simulink model "lfsr_test"  (R2021b)
settings: Solver=FixedStepAuto  StartTime=0.0  StopTime=10e-3  RelTol=1e-3
undefined symbols (not defined in the file or in its folder): hw, xc7z020clg400
libraries: hdlBasic x13, simulink x1, vmcUtilities x1
settings Model: Creator=berndorfer  LastModifiedBy=berndorfer

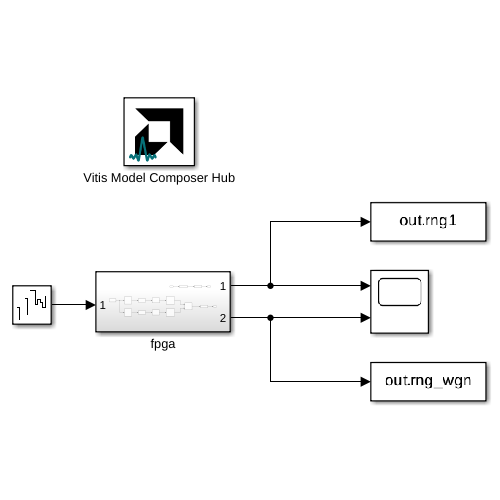
[thumbnail: Simulink's stored preview of the top-level diagram]
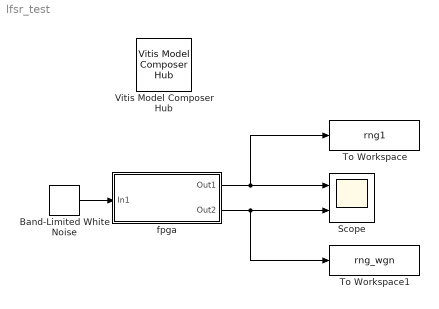
== system lfsr_test ==
  Band-Limited White Noise : simulink/Sources/Band-Limited White Noise  Cov=[2 * hw.t_s * hw.oversample]  Ts=hw.t_s*hw.oversample  seed=[23341]
  Scope : Scope  NumInputPorts=2
  To Workspace : ToWorkspace  VariableName=rng1  SaveFormat=Timeseries  SampleTime=-1
  To Workspace1 : ToWorkspace  VariableName=rng_wgn  SaveFormat=Timeseries  SampleTime=-1
  Vitis Model Composer Hub : vmcUtilities/Vitis Model Composer Hub  Tag=genX  CodeGeneration=off  SubsystemName=fpga  TargetDirectory=./code  ExportType=AI Engines  IpVendor=xilinx.com  IpLibrary=hls  IpVersion=1.0  IpHWLanguage=Verilog  AieCompilerOptions={}  AieSimulatorOptions={}  CreateTestbench=off  TestbenchStackSize=10  RunRtlSim=off  RunCSim=off  RunAieSim=off  AieSimTimeout=50000  RunAieSimProfiling=off  LaunchVitisAnalyzer=off  PlotOutput=off  RunX86Sim=off  X86SimTimeout=10  GenHwImage=off  GenLibadfXo=off  PlatformType=Not Specified  HwSystemType=Baremetal  HwValidationTarget=hw  ProjDevice=xc7z020clg400-1  ProjDevicePart=xc7z020clg400-1  AIEType=None  SamplePeriod=-1  ClockFrequency=200  DataPathParallelism=1  xilinxfamily=zynq  part=xc7z020  speed=-1  package=clg400  directory=./code/ip/fpga/src  testbench=off  incr_netlist=off  synthesis_tool=Vivado  clock_wrapper=Clock Enables  dbl_ovrd=According to Block Masks  dcm_input_clock_period=10  sysclk_period=4  simulink_period=4e-9  eval_field=0  LogFileName=''  NThreads=4
  fpga : Subsystem
  wires:
  fpga/1(Out1) -> Scope/1, To Workspace/1
  Band-Limited White Noise/1 -> fpga/1(In1)
  fpga/2(Out2) -> Scope/2, To Workspace1/1

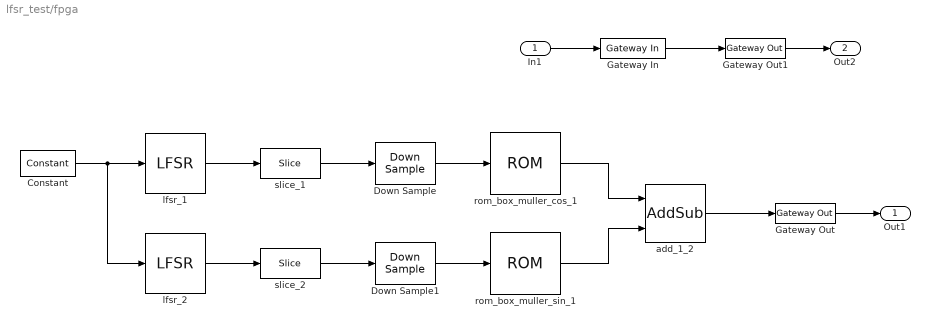
== system lfsr_test/fpga ==
  In1 : Inport
  Constant : hdlBasic/Constant  const=1.0  gui_display_data_type=Boolean  arith_type=Boolean  n_bits=16  bin_pt=14  preci_type=Single  exp_width=8  frac_width=24  explicit_period=on  period=hw.t_s*2  XmcBlockStatus=1  maskContainerNames=tabcontainer1  block_type=constant  block_config=sysgen:Constant_config
  Down Sample : hdlBasic/Down Sample  sample_ratio=hw.oversample/2  sample_phase="Last Value of Frame  (most efficient)"  en=off  rst=off  latency=1  XmcBlockStatus=1  maskContainerNames=group1  block_type=dsamp  block_config=sysgen:Downsample_config
  Down Sample1 : hdlBasic/Down Sample  sample_ratio=hw.oversample/2  sample_phase="Last Value of Frame  (most efficient)"  en=off  rst=off  latency=1  XmcBlockStatus=1  maskContainerNames=group1  block_type=dsamp  block_config=sysgen:Downsample_config
  Gateway In : hdlBasic/Gateway In  gui_display_data_type=Fixed-point  arith_type=Signed (2's comp)  n_bits=13  bin_pt=7  preci_type=Single  exp_width=8  frac_width=24  rows=1  columns=1  quantization=Truncate  overflow=Saturate  period=hw.t_s*hw.oversample  UseAsADC=off  ADCChannel='1'  interface=None  automatic_assignment=on  address_offset=hex2dec('00')  intf_name=''  intf_description=''  default_value=0  timing_constraint=None  locs_specified=off  LOCs={}  io_standard={}  inherit_from_input=off  hdl_port=on  XmcBlockStatus=1  maskContainerNames=group4  block_type=gatewayin  block_config=sysgen:gateway_in_config  block_width_w=590  block_height_w=620  block_width=640  block_height=850
  Gateway Out : hdlBasic/Gateway Out  inherit_from_input=off  hdl_port=on  rows=1  columns=1  UseAsDAC=off  DACChannel='1'  interface=None  automatic_assignment=on  address_offset=hex2dec('00')  intf_name=''  intf_description=''  timing_constraint=None  locs_specified=off  LOCs={}  io_standard={}  XmcBlockStatus=1  maskContainerNames=group4  block_type=gatewayout  block_config=sysgen:gateway_out_config  block_width_w=590  block_height_w=620  block_width=620  block_height=750
  Gateway Out1 : hdlBasic/Gateway Out  inherit_from_input=off  hdl_port=on  rows=1  columns=1  UseAsDAC=off  DACChannel='1'  interface=None  automatic_assignment=on  address_offset=hex2dec('00')  intf_name=''  intf_description=''  timing_constraint=None  locs_specified=off  LOCs={}  io_standard={}  XmcBlockStatus=1  maskContainerNames=group4  block_type=gatewayout  block_config=sysgen:gateway_out_config  block_width_w=590  block_height_w=620  block_width=620  block_height=750
  add_1_2 : hdlBasic/AddSub  mode=Addition  use_carryin=off  use_carryout=off  en=off  latency=1  precision=User Defined  arith_type="Signed  (2's comp)"  n_bits=13  bin_pt=7  quantization=Truncate  overflow=Wrap  use_behavioral_HDL=off  hw_selection=Fabric  pipelined=off  XmcBlockStatus=1  maskContainerNames=tabcontainer1  block_type=addsub  block_config=sysgen:Addsub_config
  lfsr_1 : hdlBasic/LFSR  lfsr_type=Galois  gate_type=XOR  n_bits=24  maxpolynomial=off  polynomial='c20001'  rst_value='927ce9'  rst=off  en=on  reloadable_seed=off  input_type=off  output_type=on  arith_type=Unsigned  bin_pt=0  explicit_period=off  period=1  XmcBlockStatus=1  maskContainerNames=tabcontainer1  block_type=lfsr  block_config=sysgen:LFSR_config
  lfsr_2 : hdlBasic/LFSR  lfsr_type=Galois  gate_type=XOR  n_bits=24  maxpolynomial=off  polynomial='c20001'  rst_value='6c6d84'  rst=off  en=on  reloadable_seed=off  input_type=off  output_type=on  arith_type=Unsigned  bin_pt=0  explicit_period=off  period=1  XmcBlockStatus=1  maskContainerNames=tabcontainer1  block_type=lfsr  block_config=sysgen:LFSR_config
  rom_box_muller_cos_1 : hdlBasic/ROM  depth=4096  initVector=ip.rng.box_muller_lut_cos  distributed_mem=Block RAM  rst=off  init_reg=0  en=off  latency=1  gui_display_data_type=Fixed-point  arith_type="Signed  (2's comp)"  n_bits=12  bin_pt=7  preci_type=Single  exp_width=8  frac_width=24  optimize=Area  use_rpm=on  simulation_type=fast_sim  XmcBlockStatus=1  maskContainerNames=tabcontainer1  block_type=sprom  block_config=sysgen:SPROM_config
  rom_box_muller_sin_1 : hdlBasic/ROM  depth=4096  initVector=ip.rng.box_muller_lut_sin  distributed_mem=Block RAM  rst=off  init_reg=0  en=off  latency=1  gui_display_data_type=Fixed-point  arith_type="Signed  (2's comp)"  n_bits=12  bin_pt=7  preci_type=Single  exp_width=8  frac_width=24  optimize=Area  use_rpm=on  simulation_type=fast_sim  XmcBlockStatus=1  maskContainerNames=tabcontainer1  block_type=sprom  block_config=sysgen:SPROM_config
  slice_1 : hdlBasic/Slice  nbits=12  boolean_output=off  mode=Lower Bit Location + Width  bit1=0  base1=MSB of Input  bit0=0  base0=LSB of Input  XmcBlockStatus=1  maskContainerNames=group1  block_type=slice  block_config=sysgen:Slice_config
  slice_2 : hdlBasic/Slice  nbits=12  boolean_output=off  mode=Lower Bit Location + Width  bit1=0  base1=MSB of Input  bit0=0  base0=LSB of Input  XmcBlockStatus=1  maskContainerNames=group1  block_type=slice  block_config=sysgen:Slice_config
  Out1 : Outport
  Out2 : Outport  Port=2
  wires:
  rom_box_muller_cos_1/1 -> add_1_2/1
  Constant/1 -> lfsr_2/1, lfsr_1/1
  add_1_2/1 -> Gateway Out/1
  rom_box_muller_sin_1/1 -> add_1_2/2
  Gateway Out/1 -> Out1/1
  lfsr_1/1 -> slice_1/1
  slice_1/1 -> Down Sample/1
  Down Sample/1 -> rom_box_muller_cos_1/1
  lfsr_2/1 -> slice_2/1
  slice_2/1 -> Down Sample1/1
  Down Sample1/1 -> rom_box_muller_sin_1/1
  In1/1 -> Gateway In/1
  Gateway In/1 -> Gateway Out1/1
  Gateway Out1/1 -> Out2/1
